simulink model "LQG_P2_fixed"  (R2019b)
settings: Solver=VariableStepAuto  StartTime=0.0  StopTime=50.0  RelTol=1e-3
undefined symbols (not defined in the file or in its folder): sigbuilder_block
libraries: slctrlblks x1, simulink x1
settings Model: Creator=Kevin  LastModifiedBy=Kevin

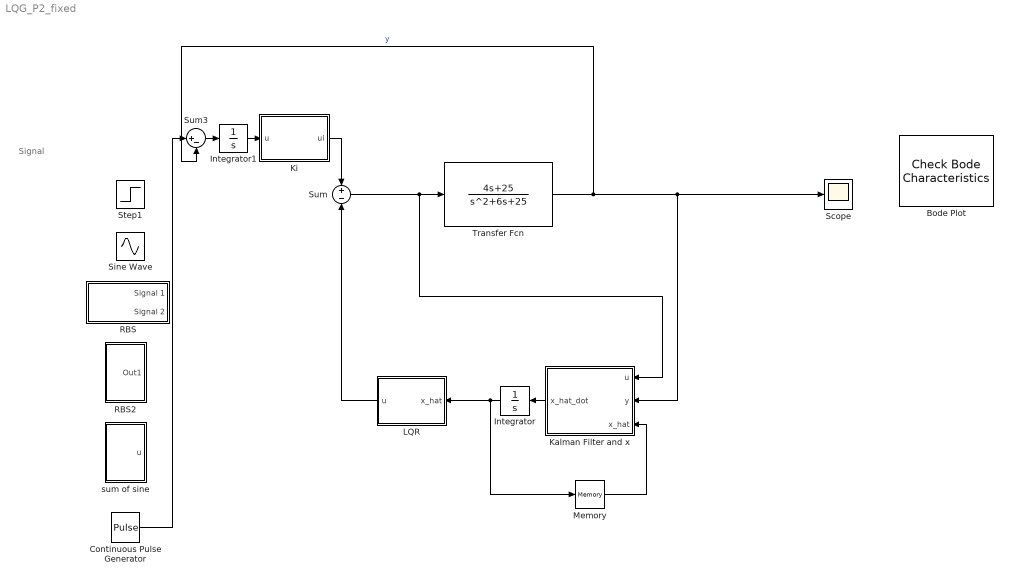
== system LQG_P2_fixed ==
  note: Signal
  Bode Plot : slctrlblks/Model Verification/Check Bode  Characteristics  InstantiateOnLoad=on  SaveOperatingPoints=off  LinearizationIOs={'/Sum', 1, 'in', 'off', '';'/Transfer Fcn', 1, 'out', 'on', ''}  LinearizeAt=SnapshotTimes  SnapshotTimes=[0]  TriggerType=rising  SampleTime=auto  RateConversionMethod=zoh  PreWarpFreq=10  UseExactDelayModel=off  UseFullBlockNameLabels=off  UseBusSignalLabels=off  enabled=on  stopWhenAssertionFail=off  export=off  ViewDlgPos=[1921 -319 1920 967.333333333333]  OpenViewOnLoad=off  LaunchViewOnOpen=off  FrequencyUnits=rad/s  MagnitudeUnits=dB  PhaseUnits=deg  TimeUnits=seconds  EnableUpperBound=off  UpperBoundFrequencies=[]  UpperBoundMagnitudes=[]  EnableLowerBound=off  LowerBoundFrequencies=[]  LowerBoundMagnitudes=[]
      settings: SourceProductName=Simulink Control Design
  Continuous Pulse Generator : DiscretePulseGenerator  PulseType=Time based  Period=1  PulseWidth=50
  Integrator : Integrator
  Integrator1 : Integrator
  Kalman Filter and x : MATLAB Function  TreatAsAtomicUnit=on
  Ki : MATLAB Function  TreatAsAtomicUnit=on
  LQR : MATLAB Function  TreatAsAtomicUnit=on
  Memory : Memory  InitialCondition=[0 0]'  InheritSampleTime=on
  "RBS " : Subsystem  Tag=STV Subsys  LoadFcn=sigbuilder_block('load');  StartFcn=sigbuilder_block('start');  StopFcn=sigbuilder_block('stop');  ClipboardFcn=sigbuilder_block('clipboard');  mask(Sigbuilder block){tuvar=[0:10]}
      mask help: Simulink:masks:SigbuilderBlock_MD
      mask init:
      | if ~strcmp(get_param(bdroot(gcbh),'SimulationStatus'),'stopped') tuvar = sigbuilder_block('maskInit'); end
      settings: CopyFcn=sigbuilder_block('copy');  DeleteFcn=sigbuilder_block('delete');  ModelCloseFcn=sigbuilder_block('modelClose');  PreSaveFcn=sigbuilder_block('preSave');  PauseFcn=sigbuilder_block('pause');  ContinueFcn=sigbuilder_block('continue');  NameChangeFcn=sigbuilder_block('namechange');  OpenFcn=sigbuilder_block('open',[215 62.5 550.5 362.5 ]);  CloseFcn=sigbuilder_block('close');
      mask Display: plot(0, 0, 100, 100,[2, 2, 32, 32, 2], [68, 8, 8, 68, 68],[32, 2], [38, 38], [32, 19, 2],[53, 60, 44], [32, 17, 17, 2],[16, 16, 31, 31]);txt = getActiveGroup(gcbh);text(2, 100, txt,'verticalAlignment', 'top');
  RBS2 : Subsystem
  Scope : Scope
  Sine Wave : Sin  Frequency=0.1  SampleTime=0
  Step1 : Step  SampleTime=0
  Sum : Sum  Inputs=+-
  Sum3 : Sum  Inputs=|+-
  Transfer Fcn : TransferFcn  Numerator=[4 25]  Denominator=[1 6 25]
  sum of sine : Subsystem
  wires:
  Transfer Fcn/1 -> Kalman Filter and x/2(y), Scope/1, Sum3/2  "y"
  Kalman Filter and x/1(x_hat_dot) -> Integrator/1
  Sum3/1 -> Integrator1/1
  Integrator1/1 -> Ki/1(u)
  LQR/1(u) -> Sum/2
  Sum/1 -> Kalman Filter and x/1(u), Transfer Fcn/1
  Integrator/1 -> Memory/1, LQR/1(x_hat)
  Continuous Pulse Generator/1 -> Sum3/1
  Memory/1 -> Kalman Filter and x/3(x_hat)
  Ki/1(ui) -> Sum/1

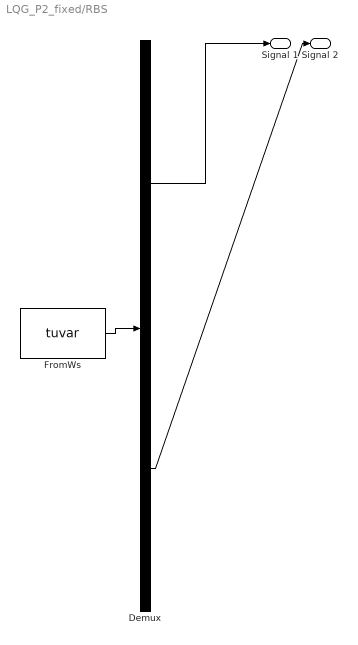
== system LQG_P2_fixed/RBS  ==
  Demux : Demux  Tag=STV Demux  Outputs=2
  FromWs : FromWorkspace  Tag=STV FromWs  VariableName=tuvar  SampleTime=0
      SigBuilderData=|
      | common.afterFinalStr = 'Extrapolate'
      | common.sampleTime = 0
      | dataSet.timeRange = [0 10]
      | dataSet.name = 'Group 1'
      | sbobj.Groups.Name = 'Group 1'
      | sbobj.Groups.Signals(1).Name = 'Signal 1'
      | sbobj.Groups.Signals(1).XData = [0 4 4 6 6 10]
      | sbobj.Groups.Signals(1).YData = [0 0 1 1 0 0]
      | sbobj.Groups.Signals(2).Name = 'Signal 2'
      | sbobj.Groups.Signals(2).XData = [0 0.2 0.2 0.3 0.3 0.5 0.5 0.7 0.7 1 1 1.1 1.1 1.3 1.3 1.4 1.4 1.5 1.5 1.7 1.7 2.1 2.1 2.2 2.2 2.7 2.7 2.8 2.8 2.9 2.9 3 3 3.1 3.1 3.5 3.5 3.7 3.7 3.8 3.8 3.9 3.9 4.2 4.2 4.4 4.4 4.7 4.7 5 5 5.1 5.1 5.3 5.3 5.6 5.6 5.7 5.7 5.8 5.8 5.9 5.9 6 6 6.1 6.1 6.2 6.2 6.7 6.7 7 7 7.1 7.1 7.2 7.2 7.3 7.3 7.4 7.4 7.5 7.5 7.8 7.8 7.9 7.9 8.1 8.1 8.5 8.5 8.6 8.6 8.8 8.8 8.9 8.9 9 9 9.2 9.2 9.5 9.5 9.6 9.6 9.7 9.7 10]
      | sbobj.Groups.Signals(2).YData = [1 1 0 0 1 1 0 0 1 1 0 0 1 1 0 0 1 1 0 0 1 1 0 0 1 1 0 0 1 1 0 0 1 1 0 0 1 1 0 0 1 1 0 0 1 1 0 0 1 1 0 0 1 1 0 0 1 1 0 0 1 1 0 0 1 1 0 0 1 1 0 0 1 1 0 0 1 1 0 0 1 1 0 0 1 1 0 0 1 1 0 0 1 1 0 0 1 1 0 0 1 1 0 0 1 1 0 0]
  Signal 1 : Outport  Tag=STV Outport
  Signal 2 : Outport  Tag=STV Outport  Port=2
  wires:
  Demux/1 -> Signal 1/1
  FromWs/1 -> Demux/1
  Demux/2 -> Signal 2/1

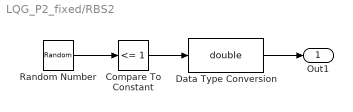
== system LQG_P2_fixed/RBS2 ==
  Compare To Constant : simulink/Logic and Bit Operations/Compare To Constant  relop=<=  const=1  OutDataTypeStr=boolean
  Data Type Conversion : DataTypeConversion  OutDataTypeStr=double
  Random Number : RandomNumber  Mean=1  SampleTime=10
  Out1 : Outport
  wires:
  Random Number/1 -> Compare To Constant/1
  Compare To Constant/1 -> Data Type Conversion/1
  Data Type Conversion/1 -> Out1/1

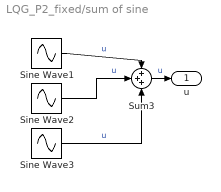
== system LQG_P2_fixed/sum of sine ==
  Sine Wave1 : Sin  Frequency=0.1  Phase=0.1  SampleTime=0
  Sine Wave2 : Sin  SampleTime=0
  Sine Wave3 : Sin  Frequency=2  SampleTime=0
  Sum3 : Sum  Inputs=+++
  u : Outport
  wires:
  Sine Wave3/1 -> Sum3/3  "u"
  Sine Wave1/1 -> Sum3/1  "u"
  Sum3/1 -> u/1  "u"
  Sine Wave2/1 -> Sum3/2  "u"

== matlab function LQG_P2_fixed/Kalman Filter and x ==
  data: u input; y input; x_hat_dot output; x_hat input
function x_hat_dot = fcn(u, y, x_hat)
coder.extrinsic("kalman","ss");
x_hat_dot = [0 0]';
L = [0 0]';
% A = [0 1; -theta(5) -theta(4)];
% B = [0 1]';
% C = [theta(3) theta(2)];
% sys = ss(A,B,C,0);

%hard coded system params
A = [0 1; -25 -6];
B = [0 1]';
C = [25 4]; 
sys = ss(A,B,C,0);

Q = 10;
R = 10;
[kalmf,L,P,M] = kalman(sys,Q,R);

x_hat_dot = A*x_hat + B*u + L*(y - C*x_hat);

== matlab function LQG_P2_fixed/LQR ==
  data: x_hat input; u output
function u = fcn(x_hat)
u = 0;
coder.extrinsic("lqr");

A = [0 1; -25 -6];
B = [0 1]';
C = [25 4]; 

%servomechanism
o = [0 0]';
A1 = [A o;C 0];
B1 = [B;0];
Q = [100 0 0; 0 100 0; 0 0 1000];
R = 0.001;
K1 = lqr(A1,B1,Q,R);
K = [K1(1) K1(2)];
u=K*x_hat;

== matlab function LQG_P2_fixed/Ki ==
  data: u input; ui output
function ui = fcn(u)
 coder.extrinsic("ss","place","matsplit",'ctrb','lqr');
% [b2, b1, b0, a1, a0] = matsplit(theta);
ui = 0;
A = [0 1; -25 -6];
B = [0 1]';
C = [25 4]; 

o = [0 0]';
A1 = [A o;C 0];
B1 = [B;0];
Q = [100 0 0; 0 100 0; 0 0 1000];
R = 0.001;

K1 = lqr(A1,B1,Q,R);
Ki = [K1(3)];
ui = Ki*u;
